simulink model "lookupTableDynamic_TestGen13"  (R2017b)
settings: Solver=FixedStepDiscrete  StartTime=0.0  StopTime=10.0  RelTol=1e-3
libraries: simulink x1
settings Model: Creator=ktrinh  LastModifiedBy=ktrinh
settings DebuggingCC: ParameterOverflowMsg=none

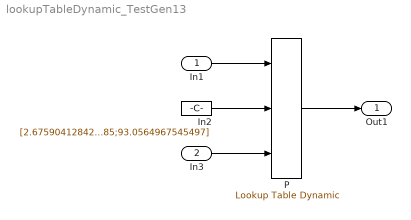
== system lookupTableDynamic_TestGen13 ==
  In1 : Inport  OutMin=0.6759  OutMax=95  OutDataTypeStr=int16  PortDimensions=1
  In3 : Inport  Port=2  PortDimensions=5
  In2 : Constant  Value=[2.67590412842418;4.29322789931548;18.8707244720968;42.2500600628885;93.0564967545497]  OutDataTypeStr=int16
  P : simulink/Lookup Tables/Lookup Table Dynamic  LookUpMeth=Interpolation-Use End Values  OutDataType=fixdt('uint8')  OutScaling=[]  OutputDataTypeScalingMode=Specify via dialog  OutDataTypeStr=uint8  RndMeth=Zero  DoSatur=on
      settings: SourceProductName=Simulink
  Out1 : Outport
  wires:
  In1/1 -> P/1
  In2/1 -> P/2
  In3/1 -> P/3
  P/1 -> Out1/1
